simulink model "Snapbot_4_leg"  (R2019b)
settings: Solver=FixedStepAuto  StartTime=0.0  StopTime=10  FixedStep=0.001  RelTol=1e-3
PreLoadFcn:
  | startup_Contact_Forces;
InitFcn:
  | SnapbotParameters;
StopFcn:
  | plot3(out.simout.data(:,1),out.simout.data(:,2),out.simout.data(:,3))
  | hold on;
  | plot3(out.simout.data(:,4),out.simout.data(:,5),out.simout.data(:,6))
  | plot3(out.simout.data(:,7),out.simout.data(:,8),out.simout.data(:,9))
  | plot3(out.simout.data(:,10),out.simout.data(:,11),out.simout.data(:,12))
  | grid on
  | grid minor
  | axis square
  | 
  | view(2)
model workspace (MATLAB code in the model file):
  other statements: smiData.RigidTransform(34).translation = [0.0 0.0 0.0];; smiData.RigidTransform(34).angle = 0.0;; smiData.RigidTransform(34).axis = [0.0 0.0 0.0];; smiData.RigidTransform(34).ID = '';; smiData.RigidTransform(1).translation = [0 0 3.5000000000000031];  % mm; smiData.RigidTransform(1).angle = 0;  % rad; smiData.RigidTransform(1).axis = [0 0 0];; smiData.RigidTransform(1).ID = 'B[Leg_Assembly_Y-P:Leg_part_01_yaw-1:-:Leg_Assembly_Y-P:v4_Hyb_X-430_IDLE_uncut-1]';; smiData.RigidTransform(2).translation = [-1.7352785874891197e-13 -35.250000000000064 1.6342482922482304e-13];  % mm; smiData.RigidTransform(2).angle = 3.1415926535897931;  % rad; smiData.RigidTransform(2).axis = [0 0.70710678118654746 0.70710678118654757];; smiData.RigidTransform(2).ID = 'F[Leg_Assembly_Y-P:Leg_part_01_yaw-1:-:Leg_Assembly_Y-P:v4_Hyb_X-430_IDLE_uncut-1]'; ... (+269)
values from neighbouring files (symbols this model uses):
  mass_xm430 = 82    [SnapbotParameters.m]
undefined symbols (not defined in the file or in its folder): smiData, X, Y, Z
libraries: sm_lib x191, nesl_utility x28, Contact_Forces_Lib x10
(part 6 of 6)

== matlab function Snapbot_4_leg/4Leg_Motion ==
  data: theta_1_1 output; theta_1_2 output; time input; theta_2_1 output; theta_2_2 output; theta_3_1 output; theta_3_2 output; theta_4_1 output; theta_4_2 output
function [theta_1_1, theta_1_2, theta_2_1, theta_2_2, theta_3_1, theta_3_2, theta_4_1, theta_4_2] = motion(time)

% Polar
theta_p = pi/3;
R = 245;
x0 = R*cos(theta_p);
y0 = R*sin(theta_p);
theta_0 = pi/3;


% Linear Motion 
x_amp = 40; % Related to forward velocity
y_amp = 30;
y_thresh = 0;
trn = 0.0; % Turning Parameter
freq = 3.5*pi;

% Yaw Rotating Motion
r_rot = 0; % Rotation Parameter 15 was successful
dir = 1; % Default 1
theta_rot = deg2rad(0);

spin_mag = deg2rad(20);
slope = atan((sin(theta_p - spin_mag) - sin(theta_p + spin_mag))/(cos(theta_p - spin_mag) - cos(theta_p + spin_mag) + 0.000001))

% Leg_1 - Left Front
x1 = (1+trn)*x_amp*sin(freq*time);
y1 = y_amp*cos(freq*time);
if y1 < y_thresh
    y1 = y_thresh;
end
x1_r = dir*r_rot*sin(freq*time);
y1_r = r_rot*cos(freq*time);
if y1_r < y_thresh
    y1_r = y_thresh;
end
x_IK_1 = x1*cos(theta_rot) - y1*sin(theta_rot) + x1_r*cos(slope) - y1_r*sin(slope) + x0;
y_IK_1 = x1*sin(theta_rot) + y1*cos(theta_rot) + x1_r*sin(slope) + y1_r*cos(slope) + y0;
[theta_1_1, theta_1_2] = IK(x_IK_1, y_IK_1 , theta_0);
% theta_2_1 = 0;
% theta_2_2 = pi;


% Leg_2
x2 = (1+trn)*x_amp*sin(freq*time + pi);
y2 = y_amp*cos(freq*time + pi);
if y2 < y_thresh
    y2 = y_thresh;
end
x2_r = dir*r_rot*sin(freq*time + pi);
y2_r = r_rot*cos(freq*time + pi);
if y2_r < y_thresh
    y2_r = y_thresh;
end
x_IK_2 = x2*cos(theta_rot) - y2*sin(theta_rot) + x2_r*cos(-slope) - y2_r*sin(-slope) - x0;
y_IK_2 = x2*sin(theta_rot) + y2*cos(theta_rot) + x2_r*sin(-slope) + y2_r*cos(-slope) + y0;
[theta_2_1, theta_2_2] = IK(x_IK_2, y_IK_2, 2*theta_0);


% theta_3_1 = 0;
% theta_3_2 = pi;

% Leg_3
x3 = (1-trn)*x_amp*sin(freq*time);
y3 = -y_amp*cos(freq*time);
if y3 > y_thresh
    y3 = y_thresh;
end
x3_r = - dir * r_rot*sin(freq*time);
y3_r = - r_rot*cos(freq*time);
if y3_r > y_thresh
    y3_r = y_thresh;
end
x_IK_3 = x3*cos(theta_rot) - y3*sin(theta_rot) + x3_r*cos(slope) - y3_r*sin(slope) - x0;
y_IK_3 = x3*sin(theta_rot) + y3*cos(theta_rot) + x3_r*sin(slope) + y3_r*cos(slope) - y0;
[theta_3_1, theta_3_2] = IK(x_IK_3, y_IK_3 , -2*theta_0);


% theta_4_1 = 0;
% theta_4_2 = pi;
% Leg_4
x4 = (1-trn)*x_amp*sin(freq*time + pi);
y4 = -y_amp*cos(freq*time + pi);
if y4 > y_thresh
    y4 = y_thresh;
end

x4_r = - dir*r_rot*sin(freq*time + pi);
y4_r = - r_rot*cos(freq*time + pi);
if y4_r > y_thresh
    y4_r = y_thresh;
end

x_IK_4 = x4*cos(theta_rot) - y4*sin(theta_rot) + x4_r*cos(-slope) - y4_r*sin(-slope) + x0;
y_IK_4 = x4*sin(theta_rot) + y4*cos(theta_rot) + x4_r*sin(-slope) + y4_r*cos(-slope) - y0;
[theta_4_1, theta_4_2] = IK(x_IK_4, y_IK_4, -theta_0);


    function [theta_1, theta_2] = IK(x,y, theta_0)
        
        L0 = 119.75;
        L1 = 56.75;
        L2 = 60;
        L3 = 90;
        L4 = 47.43;
        L5 = 25;
        L6 = 24.5;
        
        theta_offset = deg2rad(14.18);
        
        x_1 = x - L0*cos(theta_0);
        y_1 = y - L0*sin(theta_0);
        
        theta_1 = (atan2(y_1,x_1) - (theta_0));
        a = x_1 - L1*cos(theta_1 + theta_0);
        b = y_1 - L1*sin(theta_1 + theta_0);
        c = (sqrt(a^2 + b^2) - 47.5768)/60.6919;
        
        % 20th Polynomial fit
        p = [156.737295499081,632.694848125274,-262.204302436545,-3922.91183740349,-2148.52031293639,10019.1081486581,9255.93550729230,-13572.6584917378,-16000.9419544284,10449.7847280998,14885.9112089308,-4530.19976355161,-7871.87915375832,1014.49575876664,2301.83346930864,-88.7553259470797,-331.121031005098,1.65257753802370,39.5110321930851,11.1017655366948,-92.8933604502059];
        
        z = p(1)*c^20 + p(2)*c^19 + p(3)*c^18 + p(4)*c^17 + p(5)*c^16 + p(6)*c^15 + p(7)*c^14 + p(8)*c^13 + p(9)*c^12 + p(10)*c^11 + p(11)*c^10 + p(12)*c^9 + p(13)*c^8 + p(14)*c^7 + p(15)*c^6 + p(16)*c^5 + p(17)*c^4 + p(18)*c^3 + p(19)*c^2 + p(20)*c + p(21);
                
        r3 = sqrt(b^2 + z^2 + a^2);
        alpha1 = acos((L2^2 + r3^2 - L3^2)/(2*L2*r3));
        alpha2 = pi - acos(z/r3);
        theta_2 = (alpha1 + alpha2) + pi/2;
    end
end
